simulink model "controller_simulation"  (R2023b)
settings: Solver=VariableStepAuto  StartTime=0.0  StopTime=30  RelTol=1e-3
libraries: simulink x1
settings Model: Creator=tinas  LastModifiedBy=tinas

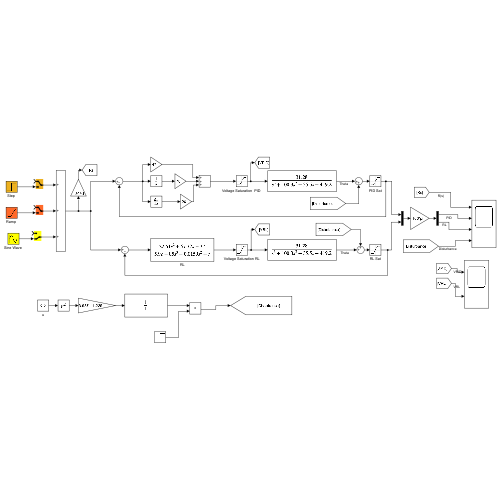
[thumbnail: Simulink's stored preview of the top-level diagram]
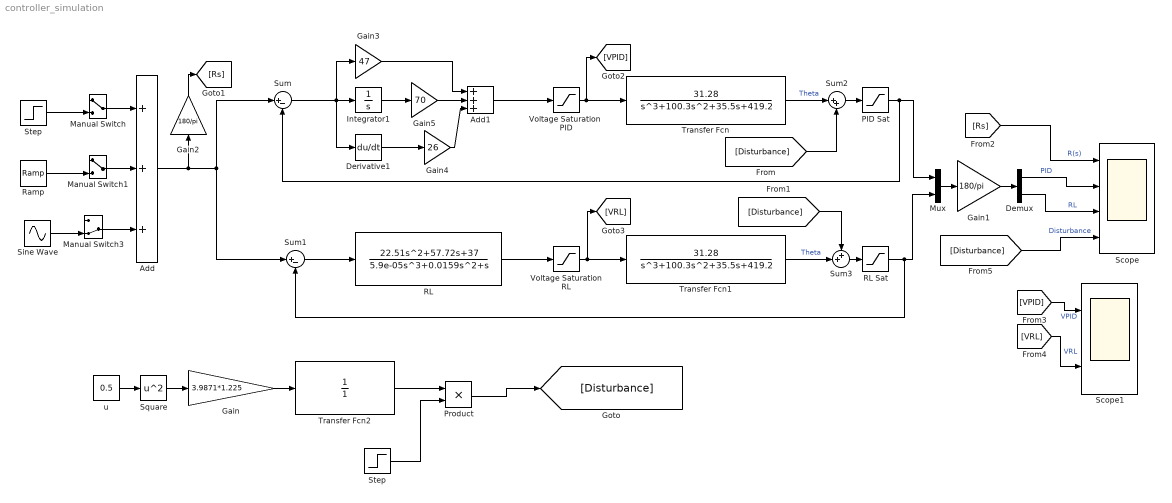
== system controller_simulation ==
  Add : Sum  Inputs=+++
  Add1 : Sum  Inputs=+++
  Demux : Demux  Outputs=2
  Derivative1 : Derivative
  Gain : Gain  Gain=3.9871*1.225
  Gain1 : Gain  Gain=180/pi
  Gain2 : Gain  Gain=180/pi
  Gain3 : Gain  Gain=47
  Gain4 : Gain  Gain=26
  Gain5 : Gain  Gain=70
  Integrator1 : Integrator
  Manual Switch : ManualSwitch
  Manual Switch1 : ManualSwitch
  Manual Switch3 : ManualSwitch  CurrentSetting=0
  Mux : Mux  Inputs=2
  PID Sat : Saturate  UpperLimit=pi/2  LowerLimit=-pi/2
  Product : Product
  RL : TransferFcn  Numerator=[22.51 57.72 37 ]  Denominator="[5.9e-05  0.0159  1 0]"
  RL Sat : Saturate  UpperLimit=pi/2  LowerLimit=-pi/2
  "Ramp " : simulink/Sources/Ramp  slope=0.01  start=0  InitialOutput=0
  Scope : Scope  NumInputPorts=4
  Scope1 : Scope  NumInputPorts=2
  "Sine Wave " : Sin  Amplitude=pi/2  SampleTime=0
  Square : Math  Operator=square
  Step : Step  Time=10  SampleTime=0
  "Step " : Step  Time=0  After=45*pi/180  SampleTime=0
  Sum : Sum  Inputs=|+-
  Sum1 : Sum  Inputs=|+-
  Sum2 : Sum  Inputs=|++
  Sum3 : Sum  Inputs=++|
  Transfer Fcn : TransferFcn  Numerator=[31.28]  Denominator="[1 100.3  35.5 419.2]"
  Transfer Fcn1 : TransferFcn  Numerator=[31.28]  Denominator="[1 100.3  35.5 419.2]"
  Transfer Fcn2 : TransferFcn  Denominator=[1]
  "Voltage Saturation  PID " : Saturate  UpperLimit=230  LowerLimit=-230
  Voltage Saturation RL : Saturate  UpperLimit=230  LowerLimit=-230
  u : Constant  Value=0.5
  wires:
  "Sine Wave "/1 -> Manual Switch3/2
  "Step "/1 -> Manual Switch/2
  Manual Switch3/1 -> Add/3
  Manual Switch1/1 -> Add/2
  "Ramp "/1 -> Manual Switch1/2
  Manual Switch/1 -> Add/1
  Add/1 -> Gain2/1, Sum1/1, Sum/1
  "Voltage Saturation  PID "/1 -> [VPID], Transfer Fcn/1
  Voltage Saturation RL/1 -> [VRL], Transfer Fcn1/1
  Add1/1 -> "Voltage Saturation  PID "/1
  Gain3/1 -> Add1/1
  Derivative1/1 -> Gain4/1
  Gain4/1 -> Add1/3
  Gain5/1 -> Add1/2
  Integrator1/1 -> Gain5/1
  Sum/1 -> Gain3/1, Derivative1/1, Integrator1/1
  RL/1 -> Voltage Saturation RL/1
  Sum1/1 -> RL/1
  u/1 -> Square/1
  Square/1 -> Gain/1
  Gain/1 -> Transfer Fcn2/1
  [Disturbance] -> Sum2/2
  [Disturbance] -> Sum3/1
  Mux/1 -> Gain1/1
  Gain2/1 -> [Rs]
  [Rs] -> Scope/1  "R(s)"
  Gain1/1 -> Demux/1
  Demux/1 -> Scope/2  "PID"
  Demux/2 -> Scope/3  "RL"
  [VRL] -> Scope1/2  "VRL"
  [VPID] -> Scope1/1  "VPID"
  [Disturbance] -> Scope/4  "Disturbance"
  Transfer Fcn2/1 -> Product/1
  Step/1 -> Product/2
  Product/1 -> [Disturbance]
  Transfer Fcn/1 -> Sum2/1  "Theta"
  Sum2/1 -> PID Sat/1
  PID Sat/1 -> Sum/2, Mux/1
  Transfer Fcn1/1 -> Sum3/2  "Theta"
  Sum3/1 -> RL Sat/1
  RL Sat/1 -> Sum1/2, Mux/2
